simulink model "pitri_FWcenterTap_Boost"  (R2021a)
settings: Solver=VariableStepAuto  StartTime=0.0  StopTime=0.1  RelTol=1e-3
libraries: spsSeriesRLCBranchLib x4, spsDiodeLib x3, spsVoltageMeasurementLib x3, spsCurrentMeasurementLib x2, spsGroundLib x2, spsRMSLib x1, spsACVoltageSourceLib x1, spsIdealSwitchLib x1, spsLinearTransformerLib x1, spsMeanLib x1, spspowerguiLib x1
settings Model: Creator=Dell  LastModifiedBy=Admin
settings SolverCC: AlgebraicLoopSolver=TrustRegion
settings DataIOCC: ReturnWorkspaceOutputs=off
settings DebuggingCC: SFMachineParentedDataDiag=warning  ArithmeticOperatorsInVariantConditions=warning
settings SFSimCC: SimUseLocalCustomCode=off  CustomCodeUndefinedFunction=UseInterfaceOnly
settings RTWCC: RTWUseLocalCustomCode=off

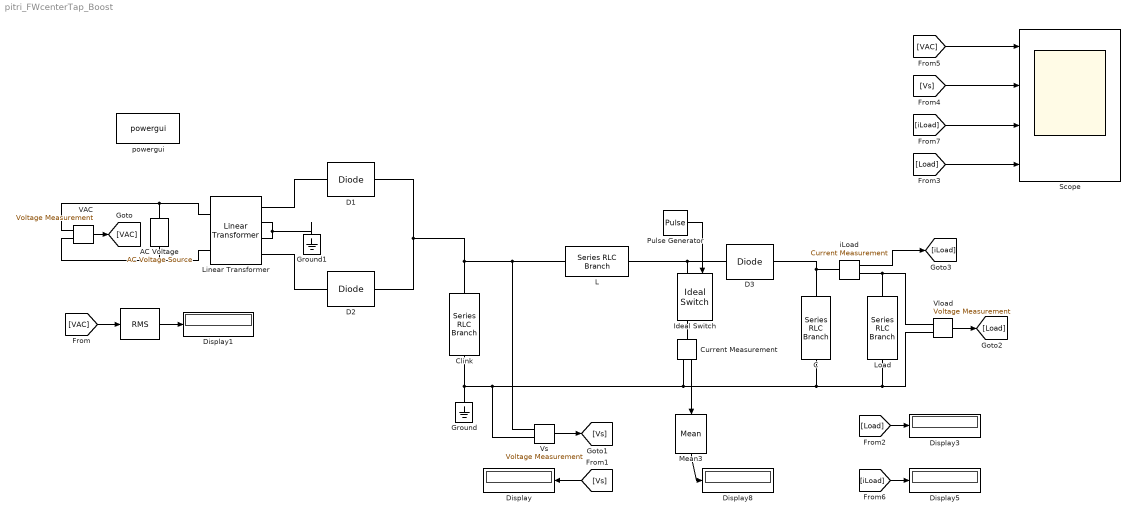
== system pitri_FWcenterTap_Boost ==
  " " : spsRMSLib/RMS  TrueRMS=on  Freq=50  RMSInit=120  Ts=0
  AC Voltage : spsACVoltageSourceLib/AC Voltage Source  Amplitude=220  Phase=0  Frequency=50  SampleTime=0  Measurements=None  BusType=swing  Pref=10e3  Qref=0  Qmin=-inf  Qmax=+inf
  C : spsSeriesRLCBranchLib/Series RLC Branch  LConnTagsString=__new0  RConnTagsString=__new0  BranchType=C  Resistance=100  Inductance=1e-3  SetiL0=off  InitialCurrent=0  Capacitance=4.3e-5  Setx0=off  InitialVoltage=0  Measurements=None
  Clink : spsSeriesRLCBranchLib/Series RLC Branch  LConnTagsString=__new0  RConnTagsString=__new0  BranchType=C  Resistance=100  Inductance=1e-3  SetiL0=off  InitialCurrent=0  Capacitance=1  Setx0=off  InitialVoltage=0  Measurements=None
  Current Measurement : spsCurrentMeasurementLib/Current Measurement  PhasorSimulation=off  OutputType=Complex  PSBequivalent=0
  D1 : spsDiodeLib/Diode  Ron=0.001  Lon=0  Vf=0.8  IC=0  UseSnubber=0  Rs=500  Cs=250e-9  Measurements=off
  D2 : spsDiodeLib/Diode  Ron=0.001  Lon=0  Vf=0.8  IC=0  UseSnubber=0  Rs=500  Cs=250e-9  Measurements=off
  D3 : spsDiodeLib/Diode  Ron=0.001  Lon=0  Vf=0.8  IC=0  UseSnubber=0  Rs=500  Cs=250e-9  Measurements=off
  Display{,1,3,5,8} (5 alike) : Display
  Ground : spsGroundLib/Ground  LConnTagsString=a
  Ground1 : spsGroundLib/Ground  LConnTagsString=a
  Ideal Switch : spsIdealSwitchLib/Ideal Switch  Ron=0.001  Lon=0  IC=0  Rs=1e5  Cs=inf  Measurements=on
  L : spsSeriesRLCBranchLib/Series RLC Branch  LConnTagsString=__new0  RConnTagsString=__new0  BranchType=L  Resistance=100  Inductance=5.181e-3  SetiL0=off  InitialCurrent=0  Capacitance=1e-6  Setx0=off  InitialVoltage=0  Measurements=None
  Linear Transformer : spsLinearTransformerLib/Linear Transformer  UNITS=pu  NominalPower=[ 250e6 50 ]  winding1="[ 1  0.02  0.08 ]"  winding2="[ 1  0.02  0.08 ]"  ThreeWindings=on  winding3=[ 1 0.02 0.08 ]  RmLm=[ 500 500 ]  Measurements=None  DataType=off
  Load : spsSeriesRLCBranchLib/Series RLC Branch  LConnTagsString=__new0  RConnTagsString=__new0  BranchType=R  Resistance=10  Inductance=1e-3  SetiL0=off  InitialCurrent=0  Capacitance=1e-6  Setx0=off  InitialVoltage=0  Measurements=None
  Mean3 : spsMeanLib/Mean  Freq=50  Vinit=0  Ts=0
  Pulse Generator : DiscretePulseGenerator  PulseType=Time based  Period=1/40000  PulseWidth=0.439*100
  Scope : Scope  NumInputPorts=4
  VAC : spsVoltageMeasurementLib/Voltage Measurement  PhasorSimulation=off  OutputType=Complex  PSBequivalent=0
  Vload : spsVoltageMeasurementLib/Voltage Measurement  PhasorSimulation=off  OutputType=Complex  PSBequivalent=0
  Vs : spsVoltageMeasurementLib/Voltage Measurement  PhasorSimulation=off  OutputType=Complex  PSBequivalent=0
  iLoad : spsCurrentMeasurementLib/Current Measurement  PhasorSimulation=off  OutputType=Complex  PSBequivalent=0
  powergui : spspowerguiLib/powergui  Priority=1  SimulationMode=Continuous  SampleTime=50e-6  frequency=60  Iterations=50  frequencyindice=50  Pbase=100e6  ErrMax=1e-4  UnitsV=kV  UnitsW=MW  buscounter=0  FunctionMessages=off  echomessages=off  EnableUseOfTLC=off  CurrentSourceSwitches=off  DisableSnubberDevices=off  DisableRonSwitches=off  DisableVfSwitches=off  DisplayEquations=off  AutomaticDiscreteSolvers=off  SolverType=Tustin/Backward Euler (TBE)  Interpol=off  ExternalGateDelay=off  methode=off  Ts=100  x0status=blocks  SPID=on  SwTol=0  HookPort=off  NonlinearTolerance=1e-4  nMaxIteration=100  ContinueOnMaxIteration=off  RestoreLinks=warning  ResistiveCurrentMeasurement=off  Frange=[0:2:500]  Ylog=off  Xlog=on  ShowGrid=off  save=off  variable=ZData  structure=0  ZoomFFT=off  StartTime=0.0  cycles=1  DisplayStyle=1  fundamental=60  FreqAxis=off  MaxFrequency=1000  frequencyindicesteady=1  RmsSteady=1  display=off
  wires:
  VAC/1 -> [VAC]
  [VAC] -> " "/1
  " "/1 -> Display1/1
  Vs/1 -> [Vs]
  [Vs] -> Display/1
  Vload/1 -> [Load]
  Pulse Generator/1 -> Ideal Switch/1
  [Load] -> Scope/4
  [VAC] -> Scope/1
  [Load] -> Display3/1
  Current Measurement/1 -> Mean3/1
  Mean3/1 -> Display8/1
  iLoad/1 -> [iLoad]
  [iLoad] -> Display5/1
  [Vs] -> Scope/2
  [iLoad] -> Scope/3
  connections:
  AC Voltage/RConn1 -- VAC/LConn1 -- Linear Transformer/LConn1
  AC Voltage/LConn1 -- VAC/LConn2 -- Linear Transformer/LConn2
  Linear Transformer/RConn1 -- D1/LConn1
  Linear Transformer/RConn4 -- D2/LConn1
  Linear Transformer/RConn2 -- Ground1/LConn1 -- Linear Transformer/RConn3
  Vs/LConn2 -- Current Measurement/RConn1 -- Vload/LConn2 -- Load/RConn1 -- C/RConn1 -- Clink/RConn1 -- Ground/LConn1
  L/RConn1 -- D3/LConn1 -- Ideal Switch/LConn1
  Load/LConn1 -- iLoad/RConn1 -- Vload/LConn1
  D3/RConn1 -- iLoad/LConn1 -- C/LConn1
  Vs/LConn1 -- L/LConn1 -- D2/RConn1 -- D1/RConn1 -- Clink/LConn1
  Current Measurement/LConn1 -- Ideal Switch/RConn1
